simulink model "sim_ekf_est_motor_4para"  (R2020b)
settings: Solver=ode1  StartTime=0.0  StopTime=100  FixedStep=0.01  RelTol=1e-3
undefined symbols (not defined in the file): DiscIntNeverNeededParam
settings Model: Creator=Admin  LastModifiedBy=ONLY-GOD

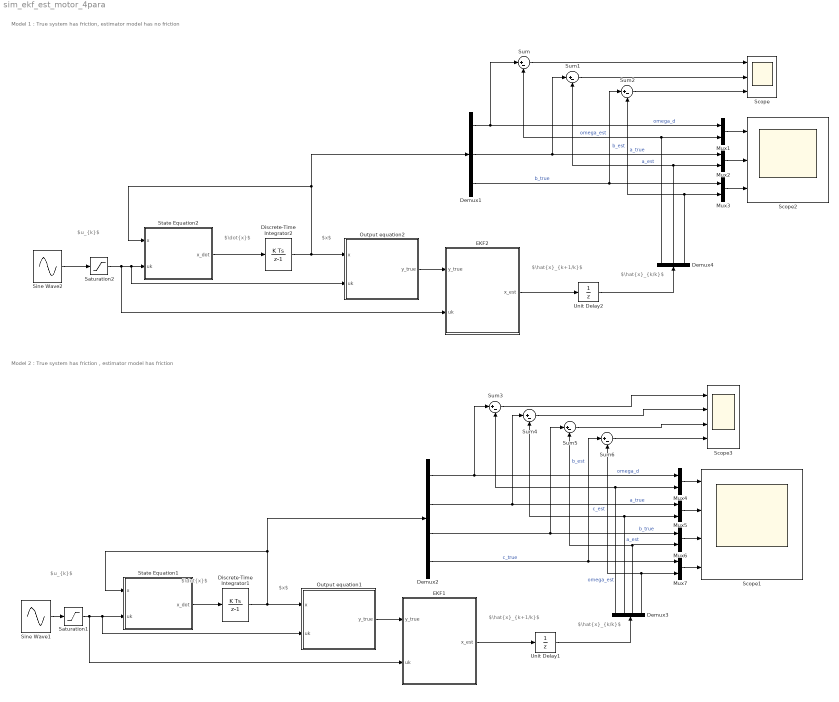
== system sim_ekf_est_motor_4para ==
  note: Model 2 : True system has friction , estimator model has friction
  note: Model 1 : True system has friction, estimator model has no friction
  note: $\dot{x}$
  note: $x$
  note: $u_{k}$
  note: $\hat{x}_{k+1/k}$
  note: $\hat{x}_{k/k}$
  note: $\dot{x}$
  note: $x$
  note: $u_{k}$
  note: $\hat{x}_{k+1/k}$
  note: $\hat{x}_{k/k}$
  Demux1 : Demux  Outputs=3
  Demux2 : Demux
  Demux3 : Demux
  Demux4 : Demux  Outputs=3
  Discrete-Time Integrator1 : DiscreteIntegrator  InitialCondition=[0;20;40;5]  SampleTime=-1  ICPrevOutput=DiscIntNeverNeededParam  ICPrevScaledInput=DiscIntNeverNeededParam
  Discrete-Time Integrator2 : DiscreteIntegrator  InitialCondition=[0;20;40]  SampleTime=-1  ICPrevOutput=DiscIntNeverNeededParam  ICPrevScaledInput=DiscIntNeverNeededParam
  EKF1 : MATLAB Function  TreatAsAtomicUnit=on
  EKF2 : MATLAB Function  TreatAsAtomicUnit=on
  Mux{1..7} (7 alike) : Mux  Inputs=2
  Output equation1 : MATLAB Function  TreatAsAtomicUnit=on
  Output equation2 : MATLAB Function  TreatAsAtomicUnit=on
  Saturation1 : Saturate  UpperLimit=24  LowerLimit=-24
  Saturation2 : Saturate  UpperLimit=24  LowerLimit=-24
  Scope : Scope  NumInputPorts=3
  Scope1 : Scope  NumInputPorts=4
  Scope2 : Scope  NumInputPorts=3
  Scope3 : Scope  NumInputPorts=4
  Sine Wave1 : Sin  Amplitude=25  Frequency=2*pi*0.1  SampleTime=0
  Sine Wave2 : Sin  Amplitude=25  Frequency=2*pi*0.1  SampleTime=0
  State Equation1 : MATLAB Function  TreatAsAtomicUnit=on
  State Equation2 : MATLAB Function  TreatAsAtomicUnit=on
  Sum{,1..6} (7 alike) : Sum  Inputs=|+-
  Unit Delay1 : UnitDelay  InitialCondition=[0;0;0;0]  SampleTime=-1  HasFrameUpgradeWarning=on
  Unit Delay2 : UnitDelay  InitialCondition=[0;0;0]  SampleTime=-1  HasFrameUpgradeWarning=on
  wires:
  Sine Wave1/1 -> Saturation1/1
  Mux7/1 -> Scope1/4
  Demux3/4 -> Mux7/2, Sum6/2  "c_est"
  Demux2/4 -> Mux7/1, Sum6/1  "c_true"
  Saturation1/1 -> EKF1/2(uk), State Equation1/2(uk), Output equation1/2(uk)
  Mux6/1 -> Scope1/3
  Mux5/1 -> Scope1/2
  Demux3/3 -> Sum5/2, Mux6/2  "b_est"
  Demux2/3 -> Mux6/1, Sum5/1  "b_true"
  Demux3/2 -> Mux5/2, Sum4/2  "a_est"
  Demux2/2 -> Mux5/1, Sum4/1  "a_true"
  Mux4/1 -> Scope1/1
  Demux3/1 -> Sum3/2, Mux4/2  "omega_est"
  Demux2/1 -> Mux4/1, Sum3/1  "omega_d"
  Unit Delay1/1 -> Demux3/1
  EKF1/1(x_est) -> Unit Delay1/1
  Output equation1/1(y_true) -> EKF1/1(y_true)
  Discrete-Time Integrator1/1 -> Output equation1/1(x), Demux2/1, State Equation1/1(x)
  State Equation1/1(x_dot) -> Discrete-Time Integrator1/1
  State Equation2/1(x_dot) -> Discrete-Time Integrator2/1
  Discrete-Time Integrator2/1 -> State Equation2/1(x), Demux1/1, Output equation2/1(x)
  Output equation2/1(y_true) -> EKF2/1(y_true)
  EKF2/1(x_est) -> Unit Delay2/1
  Unit Delay2/1 -> Demux4/1
  Demux1/1 -> Sum/1, Mux1/1  "omega_d"
  Demux4/1 -> Sum/2, Mux1/2  "omega_est"
  Mux1/1 -> Scope2/1
  Demux1/2 -> Mux2/1, Sum1/1  "a_true"
  Demux4/2 -> Mux2/2, Sum1/2  "a_est"
  Demux1/3 -> Sum2/1, Mux3/1  "b_true"
  Demux4/3 -> Sum2/2, Mux3/2  "b_est"
  Mux2/1 -> Scope2/2
  Mux3/1 -> Scope2/3
  Saturation2/1 -> EKF2/2(uk), Output equation2/2(uk), State Equation2/2(uk)
  Sine Wave2/1 -> Saturation2/1
  Sum/1 -> Scope/1
  Sum1/1 -> Scope/2
  Sum2/1 -> Scope/3
  Sum5/1 -> Scope3/3
  Sum4/1 -> Scope3/2
  Sum3/1 -> Scope3/1
  Sum6/1 -> Scope3/4

== matlab function sim_ekf_est_motor_4para/EKF2 ==
  settings: updateMethod=DISCRETE
  data: y_true input; uk input; x_est output
function x_est = ekf(y_true, uk)
Ts = 0.01;
persistent x_est_p P Qd_est R_est Qc_est;
if isempty(x_est_p)
    x_est_p = [0;0;0];
    P       = 1e-4*diag([10,1,30]);
    Qc_est  = 1e-4*diag([1,10,100]);
    Qd_est  = Ts*Qc_est;
    R_est   = 0.001;
end
c  = [1 0 0];
D  = 0;
Ck = c;
Dk = D;

%Comput Kalman Gain and update predicted value
Wk    = P*Ck'/(Ck*P*Ck'+R_est);
y_est = Ck*x_est_p+Dk*uk;
x     = x_est_p+Wk.*(y_true-y_est);

%Compute prediction at next time step
x_est = x+Ts*[-x(2)*x(1)+uk*x(3);
                          0;
                          0];

%Update error covariance matrices
P = P-Wk*Ck*P;

%Define Ak
Ak      = eye(3)+Ts*[-x(2) -x(1) uk;0 0 0;0 0 0];
P       = Ak*P*Ak'+Qd_est;
x_est_p = x_est;

== matlab function sim_ekf_est_motor_4para/Output equation2 ==
  settings: updateMethod=DISCRETE
  data: x input; uk input; y_true output
function y_true = output_eq(x,uk)
C = [1 0 0];
D = 0;
y_true = C*x+D*uk+sqrt(0.02)*randn;

== matlab function sim_ekf_est_motor_4para/State Equation2 ==
  settings: updateMethod=DISCRETE
  data: x input; uk input; x_dot output
function x_dot = state_eq(x,uk)
x_dot = [0;0;0];
x_dot(1) = -x(1)*x(2)+x(3)*uk-10*sign(x(1))*sqrt(0.01)*randn;
x_dot(2) = 0;
x_dot(3) = 0;

== matlab function sim_ekf_est_motor_4para/EKF1 ==
  settings: updateMethod=DISCRETE
  data: y_true input; uk input; x_est output
function x_est = ekf(y_true, uk)
Ts = 0.01;
persistent x_est_p P Qd_est R_est Qc_est;
if isempty(x_est_p)
    x_est_p = [0;0;0;0];
    P       = 1e-4*diag([10,1,30,10]);
    Qc_est  = 1e-4*diag([1,10,100,10]);
    Qd_est  = Ts*Qc_est;
    R_est   = 0.001;
end
c  = [1 0 0 0];
D  = 0;
Ck = c;
Dk = D;

%Comput Kalman Gain and update predicted value
Wk    = P*Ck'/(Ck*P*Ck'+R_est);
y_est = Ck*x_est_p+Dk*uk;
x     = x_est_p+Wk.*(y_true-y_est);

%Compute prediction at next time step
x_est = x+Ts*[-x(2)*x(1)+uk*x(3)-x(4)*sign(x(1));
                          0;
                          0;
                          0];

%Update error covariance matrices
P = P-Wk*Ck*P;

%Define Ak
Ak      = eye(4)+Ts*[-x(2) -x(1) uk -sign(x(1));
                 0     0    0      0;
                 0     0    0      0;
                 0     0    0      0];
P       = Ak*P*Ak'+Qd_est;
x_est_p = x_est;

== matlab function sim_ekf_est_motor_4para/Output equation1 ==
  settings: updateMethod=DISCRETE
  data: x input; uk input; y_true output
function y_true = output_eq(x,uk)
C = [1 0 0 0];
D = 0;
y_true = C*x+D*uk+sqrt(0.02)*randn;

== matlab function sim_ekf_est_motor_4para/State Equation1 ==
  settings: updateMethod=DISCRETE
  data: x input; uk input; x_dot output
function x_dot = state_eq(x,uk)
x_dot = [0;0;0;0];
x_dot(1) = -x(1)*x(2)+x(3)*uk+sqrt(0.02)-x(4)*sign(x(1))*sqrt(0.01)*randn;
x_dot(2) = 0;
x_dot(3) = 0;
x_dot(4) = 0;
